simulink model "bh_3d_pend_TEST_LINEAR_SYS_CONT_DESIGN"  (R2017a)
settings: Solver=ode45  StartTime=0.0  StopTime=45  RelTol=1e-5
undefined symbols (not defined in the file or in its folder): A, B, C, D, g, K, M_cart, m_pend, sigbuilder_block, x0
libraries: simulink_extras x4, simulink x1
settings Model: Creator=bhorton  LastModifiedBy=bhorton
settings SolverCC: ZeroCrossAlgorithm=Adaptive

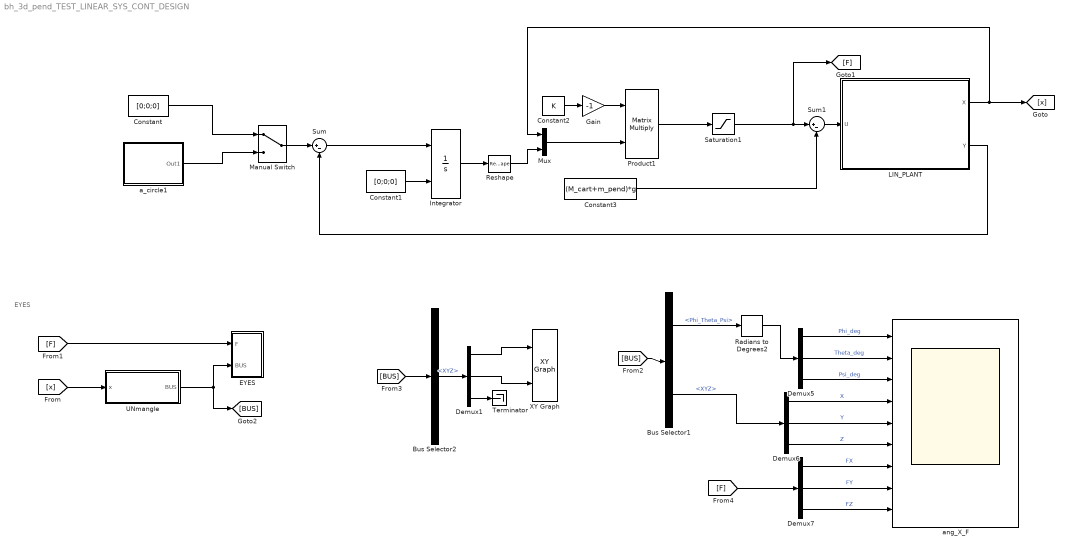
== system bh_3d_pend_TEST_LINEAR_SYS_CONT_DESIGN ==
  note: EYES
  Bus Selector1 : BusSelector  OutputSignals=Phi_Theta_Psi,XYZ
  Bus Selector2 : BusSelector  OutputSignals=XYZ
  Constant : Constant  Value=[0;0;0]  VectorParams1D=off
  Constant1 : Constant  Value=[0;0;0]  VectorParams1D=off
  Constant2 : Constant  Value=K  VectorParams1D=off
  Constant3 : Constant  Value=(M_cart+m_pend)*g  VectorParams1D=off
  Demux{1,5..7} (4 alike) : Demux  Outputs=3
  EYES : Subsystem
  Gain : Gain  Gain=-1
  Integrator : Integrator  InitialConditionSource=external
  LIN_PLANT : Subsystem
  Manual Switch : ManualSwitch
  Mux : Mux  Inputs=2
  Product1 : Product  Multiplication=Matrix(*)
  Radians to Degrees2 : simulink_extras/Transformations/Radians to Degrees
  Reshape : Reshape  OutputDimensionality=Column vector (2-D)
  Saturation1 : Saturate  UpperLimit=20  LowerLimit=-20
      settings: AttributesFormatString=|
      | MAX = %<UpperLimit>
      | MIN = %<LowerLimit>
  Sum : Sum  Inputs=|+-
  Sum1 : Sum  Inputs=|+-
  Terminator : Terminator
  UNmangle : Subsystem
  XY Graph : simulink/Sinks/XY Graph  xmin=-3  xmax=3  ymin=-3  ymax=3  st=-1
  a_circle1 : Subsystem
  ang_X_F : Scope  NumInputPorts=9
  wires:
  Constant/1 -> Manual Switch/1
  Sum/1 -> Integrator/1
  Constant1/1 -> Integrator/2
  Integrator/1 -> Reshape/1
  LIN_PLANT/1(X) -> [x], Mux/1
  Reshape/1 -> Mux/2
  Constant2/1 -> Gain/1
  Gain/1 -> Product1/1
  Mux/1 -> Product1/2
  Product1/1 -> Saturation1/1
  LIN_PLANT/2(Y) -> Sum/2
  [x] -> UNmangle/1(x)
  Sum1/1 -> LIN_PLANT/1(U)
  Constant3/1 -> Sum1/2
  Saturation1/1 -> Sum1/1, [F]
  UNmangle/1(BUS) -> [BUS], EYES/2(BUS)
  [F] -> EYES/1(F)
  Radians to Degrees2/1 -> Demux5/1
  Demux7/1 -> ang_X_F/7  "FX"
  [F] -> Demux7/1
  Bus Selector1/1 -> Radians to Degrees2/1  "<Phi_Theta_Psi>"
  Demux6/3 -> ang_X_F/6  "Z"
  Demux5/3 -> ang_X_F/3  "Psi_deg"
  Demux5/2 -> ang_X_F/2  "Theta_deg"
  Demux5/1 -> ang_X_F/1  "Phi_deg"
  Demux6/1 -> ang_X_F/4  "X"
  Demux6/2 -> ang_X_F/5  "Y"
  [BUS] -> Bus Selector1/1
  Bus Selector1/2 -> Demux6/1  "<XYZ>"
  Demux7/3 -> ang_X_F/9  "FZ"
  Demux7/2 -> ang_X_F/8  "FY"
  Manual Switch/1 -> Sum/1
  [BUS] -> Bus Selector2/1
  Bus Selector2/1 -> Demux1/1  "<XYZ>"
  Demux1/1 -> XY Graph/1
  Demux1/2 -> XY Graph/2
  a_circle1/1(Out1) -> Manual Switch/2
  Demux1/3 -> Terminator/1

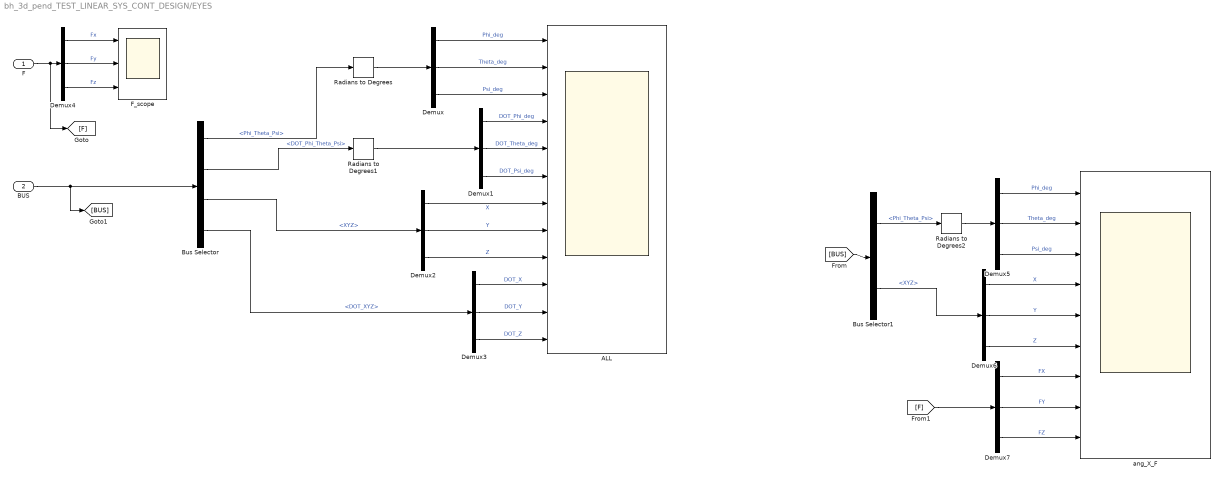
== system bh_3d_pend_TEST_LINEAR_SYS_CONT_DESIGN/EYES ==
  F : Inport
  BUS : Inport  Port=2
  ALL : Scope  NumInputPorts=12
  Bus Selector : BusSelector  OutputSignals=Phi_Theta_Psi,DOT_Phi_Theta_Psi,XYZ,DOT_XYZ
  Bus Selector1 : BusSelector  OutputSignals=Phi_Theta_Psi,XYZ
  Demux{,1..7} (8 alike) : Demux  Outputs=3
  F_scope : Scope  NumInputPorts=3
  Radians to Degrees : simulink_extras/Transformations/Radians to Degrees
  Radians to Degrees1 : simulink_extras/Transformations/Radians to Degrees
  Radians to Degrees2 : simulink_extras/Transformations/Radians to Degrees
  ang_X_F : Scope  NumInputPorts=9
  wires:
  Bus Selector/2 -> Radians to Degrees1/1  "<DOT_Phi_Theta_Psi>"
  Bus Selector/1 -> Radians to Degrees/1  "<Phi_Theta_Psi>"
  Demux4/3 -> F_scope/3  "Fz"
  Demux4/1 -> F_scope/1  "Fx"
  Demux/1 -> ALL/1  "Phi_deg"
  Radians to Degrees1/1 -> Demux1/1
  Demux3/3 -> ALL/12  "DOT_Z"
  Demux1/3 -> ALL/6  "DOT_Psi_deg"
  Bus Selector/3 -> Demux2/1  "<XYZ>"
  Demux3/1 -> ALL/10  "DOT_X"
  Demux2/3 -> ALL/9  "Z"
  Demux3/2 -> ALL/11  "DOT_Y"
  Demux2/2 -> ALL/8  "Y"
  Demux2/1 -> ALL/7  "X"
  Demux1/1 -> ALL/4  "DOT_Phi_deg"
  Demux1/2 -> ALL/5  "DOT_Theta_deg"
  Demux/2 -> ALL/2  "Theta_deg"
  BUS/1 -> [BUS], Bus Selector/1
  Demux/3 -> ALL/3  "Psi_deg"
  Bus Selector/4 -> Demux3/1  "<DOT_XYZ>"
  Radians to Degrees/1 -> Demux/1
  Demux4/2 -> F_scope/2  "Fy"
  F/1 -> [F], Demux4/1
  Demux7/2 -> ang_X_F/8  "FY"
  Bus Selector1/2 -> Demux6/1  "<XYZ>"
  Demux6/2 -> ang_X_F/5  "Y"
  [BUS] -> Bus Selector1/1
  Demux7/3 -> ang_X_F/9  "FZ"
  Demux6/3 -> ang_X_F/6  "Z"
  Bus Selector1/1 -> Radians to Degrees2/1  "<Phi_Theta_Psi>"
  Demux5/1 -> ang_X_F/1  "Phi_deg"
  Demux5/2 -> ang_X_F/2  "Theta_deg"
  Demux5/3 -> ang_X_F/3  "Psi_deg"
  Demux6/1 -> ang_X_F/4  "X"
  Radians to Degrees2/1 -> Demux5/1
  Demux7/1 -> ang_X_F/7  "FX"
  [F] -> Demux7/1

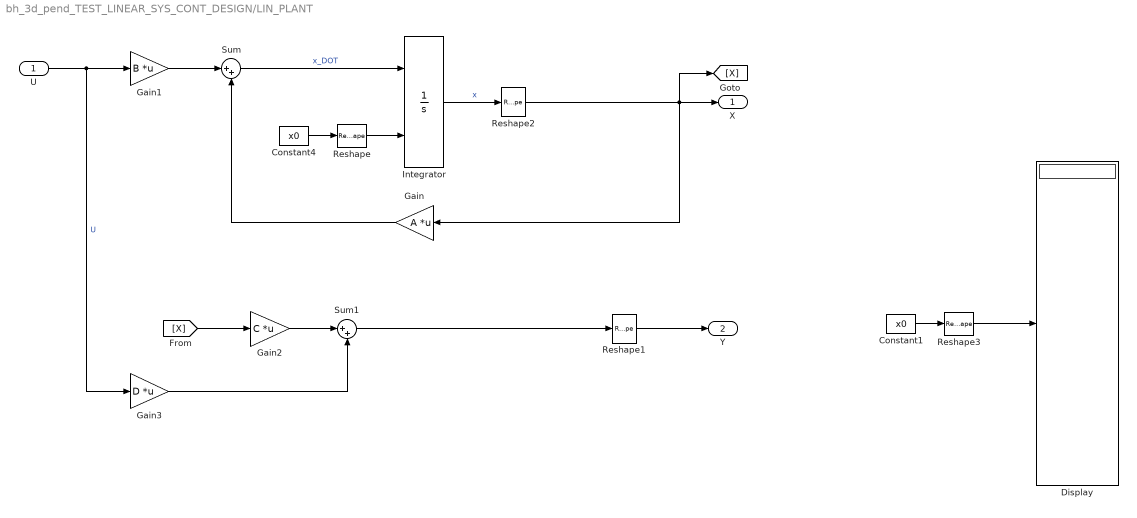
== system bh_3d_pend_TEST_LINEAR_SYS_CONT_DESIGN/LIN_PLANT ==
  U : Inport
  Constant1 : Constant  Value=x0
  Constant4 : Constant  Value=x0
  Display : Display
  Gain : Gain  Gain=A  Multiplication=Matrix(K*u)
  Gain1 : Gain  Gain=B  Multiplication=Matrix(K*u)
  Gain2 : Gain  Gain=C  Multiplication=Matrix(K*u)
  Gain3 : Gain  Gain=D  Multiplication=Matrix(K*u)
  Integrator : Integrator  InitialConditionSource=external
  Reshape{,1..3} (4 alike) : Reshape  OutputDimensionality=Column vector (2-D)
  Sum : Sum  Inputs=|++
  Sum1 : Sum  Inputs=|++
  X : Outport
  Y : Outport  Port=2
  wires:
  Reshape/1 -> Integrator/2
  Constant4/1 -> Reshape/1
  Sum/1 -> Integrator/1  "x_DOT"
  U/1 -> Gain3/1, Gain1/1  "U"
  Gain1/1 -> Sum/1
  Integrator/1 -> Reshape2/1  "x"
  Sum1/1 -> Reshape1/1
  Reshape2/1 -> [X], X/1, Gain/1
  Reshape1/1 -> Y/1
  Constant1/1 -> Reshape3/1
  Reshape3/1 -> Display/1
  Gain/1 -> Sum/2
  [X] -> Gain2/1
  Gain2/1 -> Sum1/1
  Gain3/1 -> Sum1/2

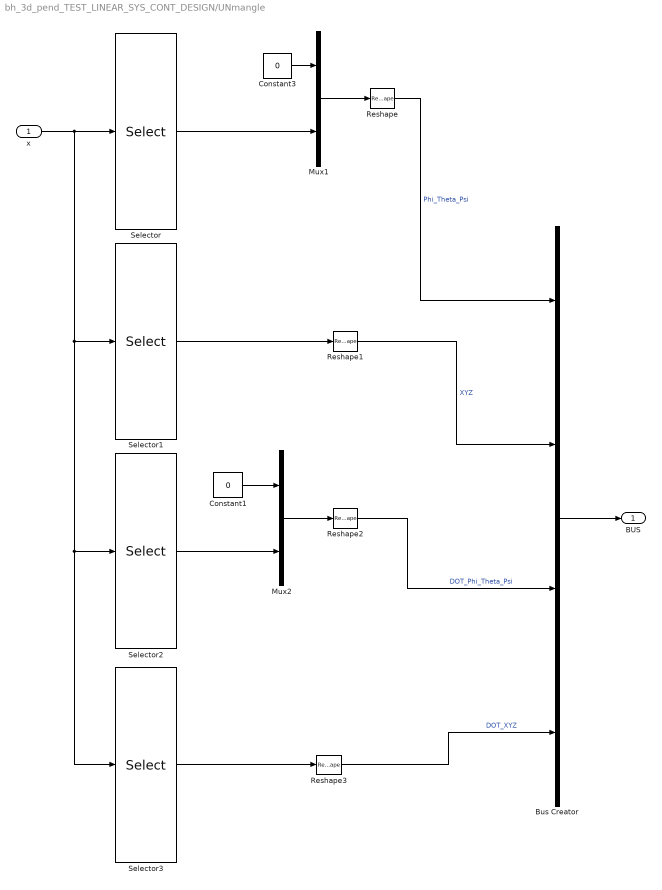
== system bh_3d_pend_TEST_LINEAR_SYS_CONT_DESIGN/UNmangle ==
  x : Inport
  Bus Creator : BusCreator  Inputs=4
  Constant1 : Constant  Value=0  VectorParams1D=off
  Constant3 : Constant  Value=0  VectorParams1D=off
  Mux1 : Mux  Inputs=2
  Mux2 : Mux  Inputs=2
  Reshape{,1..3} (4 alike) : Reshape  OutputDimensionality=Column vector (2-D)
  Selector : Selector  InputPortWidth=10  IndexOptions=Index vector (dialog)  Indices=[1,2]  OutputSizes=1
  Selector1 : Selector  InputPortWidth=10  IndexOptions=Index vector (dialog)  Indices=3:5  OutputSizes=1
  Selector2 : Selector  InputPortWidth=10  IndexOptions=Index vector (dialog)  Indices=6:7  OutputSizes=1
  Selector3 : Selector  InputPortWidth=10  IndexOptions=Index vector (dialog)  Indices=8:10  OutputSizes=1
  BUS : Outport
  wires:
  x/1 -> Selector3/1, Selector2/1, Selector1/1, Selector/1
  Constant3/1 -> Mux1/1
  Selector/1 -> Mux1/2
  Mux1/1 -> Reshape/1
  Selector1/1 -> Reshape1/1
  Selector2/1 -> Mux2/2
  Constant1/1 -> Mux2/1
  Mux2/1 -> Reshape2/1
  Selector3/1 -> Reshape3/1
  Bus Creator/1 -> BUS/1
  Reshape/1 -> Bus Creator/1  "Phi_Theta_Psi"
  Reshape1/1 -> Bus Creator/2  "XYZ"
  Reshape2/1 -> Bus Creator/3  "DOT_Phi_Theta_Psi"
  Reshape3/1 -> Bus Creator/4  "DOT_XYZ"

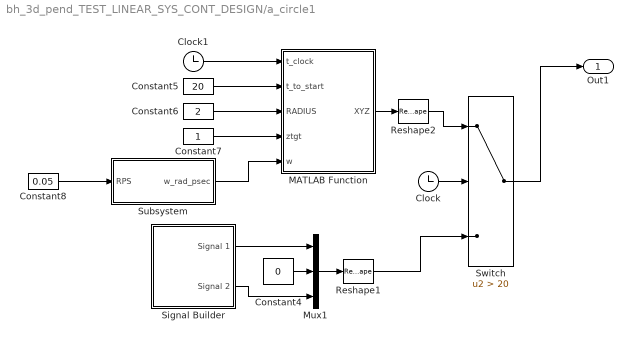
== system bh_3d_pend_TEST_LINEAR_SYS_CONT_DESIGN/a_circle1 ==
  Clock : Clock
  Clock1 : Clock
  Constant4 : Constant  Value=0  VectorParams1D=off
  Constant5 : Constant  Value=20  VectorParams1D=off
  Constant6 : Constant  Value=2  VectorParams1D=off
  Constant7 : Constant  VectorParams1D=off
  Constant8 : Constant  Value=0.05  VectorParams1D=off
  MATLAB Function : MATLAB Function  TreatAsAtomicUnit=on
  Mux1 : Mux  Inputs=3
  Reshape1 : Reshape  OutputDimensionality=Column vector (2-D)
  Reshape2 : Reshape  OutputDimensionality=Column vector (2-D)
  Signal Builder : Subsystem  Tag=STV Subsys  LoadFcn=sigbuilder_block('load');  StartFcn=sigbuilder_block('start');  StopFcn=sigbuilder_block('stop');  ClipboardFcn=sigbuilder_block('clipboard');  mask(Sigbuilder block){tuvar=[0:10]}
      mask help: Simulink:masks:SigbuilderBlock_MD
      mask init:
      | if ~strcmp(get_param(bdroot(gcbh),'SimulationStatus'),'stopped') tuvar = sigbuilder_block('maskInit'); end
      settings: CopyFcn=sigbuilder_block('copy');  DeleteFcn=sigbuilder_block('delete');  ModelCloseFcn=sigbuilder_block('modelClose');  PreSaveFcn=sigbuilder_block('preSave');  PauseFcn=sigbuilder_block('pause');  ContinueFcn=sigbuilder_block('continue');  NameChangeFcn=sigbuilder_block('namechange');  OpenFcn=sigbuilder_block('open',[437.6 199.2 550.4 400 ]);  CloseFcn=sigbuilder_block('close');
      mask Display: plot(0, 0, 100, 100,[2, 2, 32, 32, 2], [68, 8, 8, 68, 68],[32, 2], [38, 38], [32, 19, 2],[53, 60, 44], [32, 17, 17, 2],[16, 16, 31, 31]);txt = getActiveGroup(gcbh);text(2, 100, txt,'verticalAlignment', 'top');
  Subsystem : Subsystem
  Switch : Switch  Criteria=u2 > Threshold  Threshold=20
  Out1 : Outport
  wires:
  Switch/1 -> Out1/1
  MATLAB Function/1(XYZ) -> Reshape2/1
  Constant6/1 -> MATLAB Function/3(RADIUS)
  Constant7/1 -> MATLAB Function/4(ztgt)
  Subsystem/1(w_rad_psec) -> MATLAB Function/5(w)
  Constant5/1 -> MATLAB Function/2(t_to_start)
  Reshape1/1 -> Switch/3
  Constant4/1 -> Mux1/2
  Signal Builder/1(Signal 1) -> Mux1/1
  Signal Builder/2(Signal 2) -> Mux1/3
  Mux1/1 -> Reshape1/1
  Clock/1 -> Switch/2
  Clock1/1 -> MATLAB Function/1(t_clock)
  Constant8/1 -> Subsystem/1(RPS)
  Reshape2/1 -> Switch/1

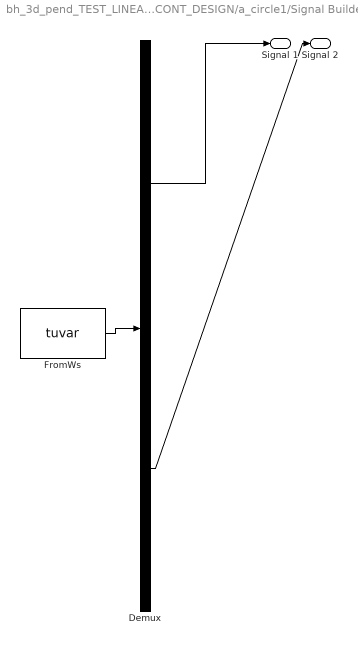
== system bh_3d_pend_TEST_LINEAR_SYS_CONT_DESIGN/a_circle1/Signal Builder ==
  Demux : Demux  Tag=STV Demux  Outputs=2
  FromWs : FromWorkspace  Tag=STV FromWs  VariableName=tuvar  SampleTime=0
      SigBuilderData=|
      | common.afterFinalStr = 'Extrapolate'
      | common.sampleTime = 0
      | dataSet.timeRange = [0 22]
      | dataSet.name = 'Group 1'
      | sbobj.Groups.Name = 'Group 1'
      | sbobj.Groups.Signals(1).Name = 'Signal 1'
      | sbobj.Groups.Signals(1).XData = [0 7.95 7.95 22]
      | sbobj.Groups.Signals(1).YData = [0 0 1.99 1.98]
      | sbobj.Groups.Signals(2).Name = 'Signal 2'
      | sbobj.Groups.Signals(2).XData = [0 12 16 22]
      | sbobj.Groups.Signals(2).YData = [0 0 1 1]
      | sbobj.Groups.TimeRange = [0 22]
  Signal 1 : Outport  Tag=STV Outport
  Signal 2 : Outport  Tag=STV Outport  Port=2
  wires:
  Demux/1 -> Signal 1/1
  FromWs/1 -> Demux/1
  Demux/2 -> Signal 2/1

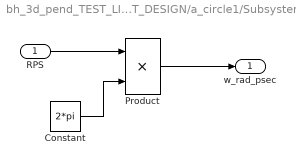
== system bh_3d_pend_TEST_LINEAR_SYS_CONT_DESIGN/a_circle1/Subsystem ==
  RPS : Inport
  Constant : Constant  Value=2*pi
  Product : Product  Inputs=**
  w_rad_psec : Outport
  wires:
  Constant/1 -> Product/2
  RPS/1 -> Product/1
  Product/1 -> w_rad_psec/1

== matlab function bh_3d_pend_TEST_LINEAR_SYS_CONT_DESIGN/a_circle1/MATLAB Function ==
  data: t_clock input; XYZ output; t_to_start input; RADIUS input; ztgt input; w input
function XYZ = fcn(t_clock, t_to_start, RADIUS, ztgt, w)

t    = t_clock - t_to_start;

theta = w*t;

x = RADIUS * cos(theta);
y = RADIUS * sin(theta);
z = ztgt;


XYZ = [x;y;z];
